simulink model "StateDiagram4"  (R2025b)
settings: Solver=VariableStepAuto  StartTime=0.0  StopTime=Inf  RelTol=1e-3
libraries: simulink_extras x1
settings Model: Creator=Soochan Kim  LastModifiedBy=Soochan Kim

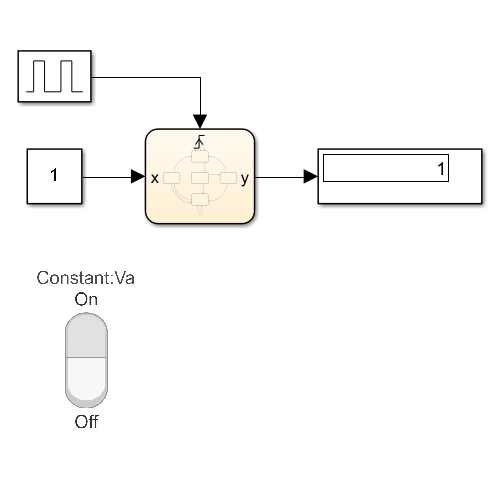
[thumbnail: Simulink's stored preview of the top-level diagram]
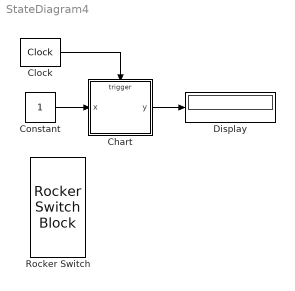
== system StateDiagram4 ==
  Chart : Stateflow chart  TreatAsAtomicUnit=on
  Clock : simulink_extras/Flip Flops/Clock  period=2
  Constant : Constant
  Display : Display
  Rocker Switch : RockerSwitchBlock
  wires:
  Constant/1 -> Chart/1(x)
  Chart/1(y) -> Display/1
  Clock/1 -> Chart/Trigger

== stateflow chart StateDiagram4/Chart ==
  settings: executeAtInitialization=1
  state S0
  state S02
  state S04
  state S01
  state S03
  S0 -> S0 [order 2] : [x==0]{y=0}
  (default) -> S0
  S02 -> S0 [order 2] : [x==0]{y=0}
  S01 -> S0 [order 2] : [x==0]{y=0}
  S0 -> S04 [order 1] : [x==1]{y=0}
  S04 -> S01 [order 1] : [x==0]{y=0}
  S02 -> S03 [order 1] : [x==1]{y=1}
  S03 -> S02 [order 1] : [x==0]{y=0}
  S04 -> S03 [order 2] : [x==1]{y=0}
  S01 -> S03 [order 1] : [x==1]{y=0}
  S03 -> S03 [order 2] : [x==1]{y=1}
  data: x input; y output
  events: clk input RISING_EDGE_EVENT
